simulink model "CM510A_MotAg3Meas"  (R2013b)
settings: Solver=FixedStepDiscrete  SolverMode=SingleTasking  StartTime=0.0  StopTime=1  FixedStep=0.0000625  RelTol=1e-3
values from neighbouring files (symbols this model uses):
  MOTAGCNTRREGMASK_CNT_U16 = DataDict.Constant    [CM510A_MotAg3Meas_DataDict.m]
  MOTAGLIM_CNT_U16 = DataDict.Constant    [CM510A_MotAg3Meas_DataDict.m]
undefined symbols (not defined in the file or in its folder): sigbuilder_block
libraries: simulink x4, NexteerUtilities x1
settings Model: RequirementInfo="{}  %GIDa_ca294f38_ed7c_4fb9_8c54_f4d56271bfc7"  ModifiedHistory=Rev 008: Updated model to Matlab 2013B, added comments to show requirement linkage  PauseTimes=0.5  Creator=nz3zln  LastModifiedBy=TZ8CY0
settings SolverCC: AutoInsertRateTranBlk=on  InsertRTBMode=Always
settings DataIOCC: LimitDataPoints=off  SaveFormat=Structure  ReturnWorkspaceOutputs=on
settings OptimizationCC: BlockReduction=off  InlineParams=on  ZeroExternalMemoryAtStartup=off  ZeroInternalMemoryAtStartup=off  OptimizeModelRefInitCode=on  LifeSpan=1
settings DebuggingCC: SignalInfNanChecking=error  SignalRangeChecking=warning  UnderspecifiedInitializationDetection=Simplified  SolverPrmCheckMsg=error  InheritedTsInSrcMsg=error  DiscreteInheritContinuousMsg=error  SingleTaskRateTransMsg=error  TasksWithSamePriorityMsg=error  SigSpecEnsureSampleTimeMsg=error  CheckMatrixSingularityMsg=error  ParameterUnderflowMsg=error  ParameterPrecisionLossMsg=error  ParameterTunabilityLossMsg=error  FixptConstUnderflowMsg=warning  FixptConstOverflowMsg=warning  VectorMatrixConversionMsg=error  SignalLabelMismatchMsg=error  UnconnectedInputMsg=error  UnconnectedOutputMsg=error  UnconnectedLineMsg=error  SFcnCompatibilityMsg=error  UniqueDataStoreMsg=warning  BusObjectLabelMismatch=error  RootOutportRequireBusObject=error  AssertControl=DisableAll  ModelReferenceIOMsg=error  ModelReferenceVersionMismatchMessage=warning  ModelReferenceIOMismatchMessage=error  ModelReferenceCSMismatchMessage=warning  ModelReferenceDataLoggingMessage=error  StateNameClashWarn=warning  StrictBusMsg=ErrorOnBusTreatedAsVector  NonBusSignalsTreatedAsBus=error  SFUnexpectedBacktrackingDiag=error  SFInvalidInputDataAccessInChartInitDiag=error  SFNoUnconditionalDefaultTransitionDiag=error  SFTransitionOutsideNaturalParentDiag=error  SFUnconditionalTransitionShadowingDiag=error  SFUndirectedBroadcastEventsDiag=error
settings ModelReferenceCC: ModelReferenceNumInstancesAllowed=Single
settings RTWCC: SystemTargetFile=autosar.tlc  GenCodeOnly=on  TemplateMakefile=ert_default_tmf  Description=AUTOSAR  GenerateReport=on  ProcessScript=autosar_make_rtw_hook  LaunchReport=on
settings CodeAppCC: GenerateComments=off  IgnoreCustomStorageClasses=off  CustomSymbolStrType=$N$R$M  CustomSymbolStrBlkIO=$N$M  SimulinkBlockComments=off
settings STFCustomTargetCC: ParMdlRefBuildCompliant=on  CompOptLevelCompliant=on  IncludeMdlTerminateFcn=off  CombineOutputUpdateFcns=on  SuppressErrorStatus=on  ERTFirstTimeCompliant=on  ERTCustomFileBanners=on  SupportNonFinite=off  SupportComplex=off  SupportContinuousTime=off  SupportNonInlinedSFcns=off  MATLABClassNameForMDSCustomization=Simulink.SoftwareTarget.ERTCustomization  AutosarCompliant=on  GRTInterface=off  SystemTargetFile=autosar.tlc
settings ERTTargetCC: CodeReplacementLibrary=ANSI_C  ConcurrentExecutionCompliant=off  IncludeMdlTerminateFcn=off  SuppressErrorStatus=on  SupportNonFinite=off  SupportComplex=off  ModelStepFunctionPrototypeControlCompliant=off  CPPClassGenCompliant=off  AutosarCompliant=on  InlinedParameterPlacement=NonHierarchical  ERTCustomFileTemplate=example_file_process.tlc  EnableUserReplacementTypes=on

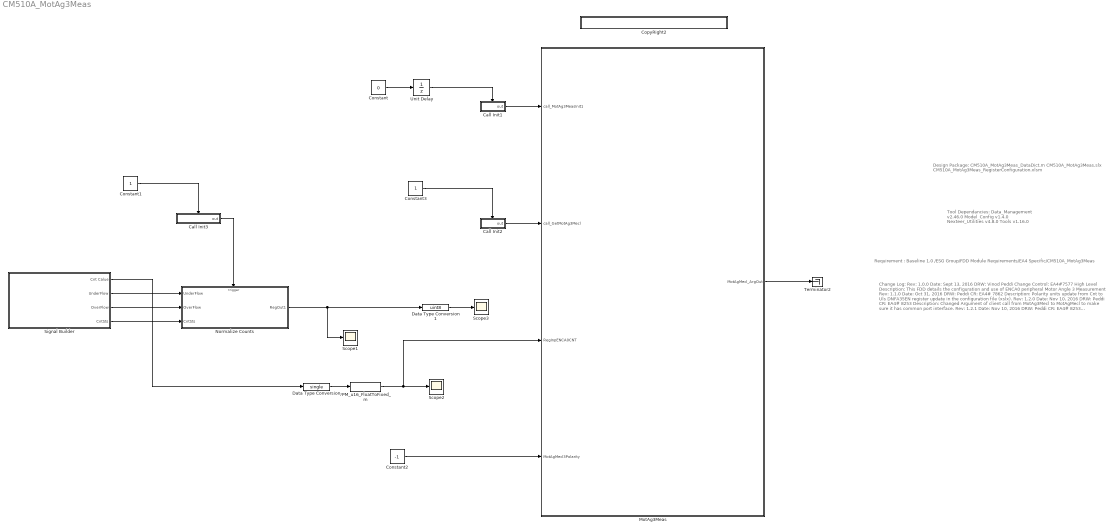
== system CM510A_MotAg3Meas ==
  note: Requirement : Baseline 1.0
      | /ESG Group/FDD Module Requirements/EA4 Specific/CM510A_MotAg3Meas
  note: Tool Dependancies:
      | Data_Management v2.46.0
      | Model_Config v1.4.0
      | Nexteer_Utilities v4.8.0
      | Tools v1.16.0
  note: Design Package:
      | CM510A_MotAg3Meas_DataDict.m
      | CM510A_MotAg3Meas.slx
      | CM510A_MotAg3Meas_RegisterConfiguration.xlsm
  note: Change Log:
      |
      | Rev: 1.0.0
      | Date: Sept 13, 2016
      | DRW: Vinod Peddi
      | Change Control: EA4#7577
      | High Level Description:
      | This FDD details the configuration and use of ENCA0 peripheral Motor Angle 3 Measurement
      |
      | Rev: 1.1.0
      | Date: Oct 31, 2016
      | DRW: Peddi
      | CR: EA4# 7862
      | Description: Polarity units update from Cnt to Uls
      | DNFA35EN register update in the configuration file (xslx).
      |
      | Rev: 1.2.0
      | Date: Nov 10, 2016
      | DRW: Peddi
      | CR: EA4# 8253
      | Description: Changed Argument of client call from MotAg3Mecl to MotAgMecl to
      | make sure it has common port interface.
      |
      | Rev: 1.2.1
      | Date: Nov 10, 2016
      | DRW: Peddi
      | CR: EA4# 8253
      | Description: Removed PIC and Noise Filter Config. (Will be handled by CM10)
  Call Init1 : Subsystem  TreatAsAtomicUnit=on
  Call Init2 : Subsystem  TreatAsAtomicUnit=on
  Call Init3 : Subsystem  TreatAsAtomicUnit=on
  Constant : Constant  Value=0  OutDataTypeStr=uint8
  Constant1 : Constant  OutDataTypeStr=int8
  Constant2 : Constant  Value=-1  OutDataTypeStr=int8
  Constant3 : Constant  OutDataTypeStr=int8
  CopyRight2 : Subsystem  Description=|  mask(Copyright Information){none=on}
      | Copyright info block.                                               
      |                                                                     
      | Place copyright information at the top of every subsystem in design.
      mask prompts: none "No parameters"
      mask help: Place copyright information at the top of every subsystem in design.
      mask Display:
      | NxtrConf = 'Nexteer Confidential';
      | 
      | sys = bdroot; %handle for the current model ("system")
      | first = get_param(sys,'Created');
      | first = first(end-3:end);  %year is last four digits
      | 
      | last = get_param(sys,'LastModifiedDate');
      | if isempty(last)
      |     last = datestr(now,'yyyy');
      | else
      |     last = last(end-3:end);
      | end
      | 
      | if strcmp(first,last)
      |     fprintf('%s -- Copyright %s Nexteer',NxtrConf,first)
      | else
      |     fprintf('%s -- %s%s- %s Nexteer',NxtrConf,char(169),first,last)
      | end
  Data Type Conversion : DataTypeConversion  OutDataTypeStr=single
  Data Type Conversion1 : DataTypeConversion  OutDataTypeStr=uint8
  FPM_u16_FloatToFixed_m : NexteerUtilities/Fixed Point Math Conversions/FPM_u16_FloatToFixed_m  SFunctionSpec=uint16 y1 = FPM_u16_FloatToFixed_m(single u1, single p1)  Param1=16
      settings: AttributesFormatString=u16_FloatToFixed
  MotAg3Meas : Subsystem
  Normalize Counts : Subsystem
  Scope1 : Scope
  Scope2 : Scope
      settings: SaveName=ScopeData7
  Scope3 : Scope
  Signal Builder : Subsystem  Tag=STV Subsys  LoadFcn=sigbuilder_block('load');  StartFcn=sigbuilder_block('start');  StopFcn=sigbuilder_block('stop');  ClipboardFcn=sigbuilder_block('clipboard');  mask(Sigbuilder block){}
      mask help: Simulink:masks:SigbuilderBlock_MD
      mask init:
      | if ~strcmp(get_param(bdroot(gcbh),'SimulationStatus'),'stopped') tuvar = sigbuilder_block('maskInit'); end
      settings: CopyFcn=sigbuilder_block('copy');  DeleteFcn=sigbuilder_block('delete');  ModelCloseFcn=sigbuilder_block('modelClose');  PreSaveFcn=sigbuilder_block('preSave');  PauseFcn=sigbuilder_block('pause');  ContinueFcn=sigbuilder_block('continue');  NameChangeFcn=sigbuilder_block('namechange');  OpenFcn=sigbuilder_block('open',[0 30 1440 723 ]);  CloseFcn=sigbuilder_block('close');
      mask Display: plot(0, 0, 100, 100,[2, 2, 32, 32, 2], [68, 8, 8, 68, 68],[32, 2], [38, 38], [32, 19, 2],[53, 60, 44], [32, 17, 17, 2],[16, 16, 31, 31]);txt = getActiveGroup(gcbh);text(2, 100, txt,'verticalAlignment', 'top');
  Terminator2 : Terminator
  Unit Delay : UnitDelay  InitialCondition=1  SampleTime=-1
  wires:
  Constant/1 -> Unit Delay/1
  Unit Delay/1 -> Call Init1/Enable
  Constant3/1 -> Call Init2/Enable
  Call Init1/1(out) -> MotAg3Meas/1(call_MotAg3MeasInit1)
  Call Init2/1(out) -> MotAg3Meas/2(call_GetMotAg3Mecl)
  FPM_u16_FloatToFixed_m/1 -> MotAg3Meas/3(RegInpENCA0CNT), Scope2/1
  Normalize Counts/1(RegOut1) -> Data Type Conversion1/1, Scope1/1
  MotAg3Meas/1(MotAgMecl_ArgOut) -> Terminator2/1
  Data Type Conversion/1 -> FPM_u16_FloatToFixed_m/1
  Constant1/1 -> Call Init3/Enable
  Call Init3/1(out) -> Normalize Counts/Trigger
  Signal Builder/1(Cnt Calue) -> Data Type Conversion/1
  Signal Builder/2(UnderFlow) -> Normalize Counts/1(UnderFlow)
  Signal Builder/3(OverFlow) -> Normalize Counts/2(OverFlow)
  Signal Builder/4(CntSts) -> Normalize Counts/3(CntSts)
  Data Type Conversion1/1 -> Scope3/1
  Constant2/1 -> MotAg3Meas/4(MotAgMecl3Polarity)

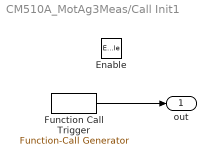
== system CM510A_MotAg3Meas/Call Init1 ==
  Enable : EnablePort
  Function Call Trigger : simulink/Ports & Subsystems/Function-Call Generator  RequirementInfo={} %GIDa_b7229461_487a_40de_bfdf_dab388053d82  sample_time=0.002  numberOfIterations=1
  out : Outport
  wires:
  Function Call Trigger/1 -> out/1

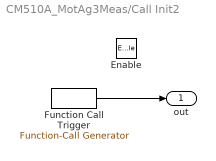
== system CM510A_MotAg3Meas/Call Init2 ==
  Enable : EnablePort
  Function Call Trigger : simulink/Ports & Subsystems/Function-Call Generator  RequirementInfo={} %GIDa_a0a97c4f_3e8f_431b_a781_191ff84f73ef  sample_time=0.0005  numberOfIterations=1
  out : Outport
  wires:
  Function Call Trigger/1 -> out/1

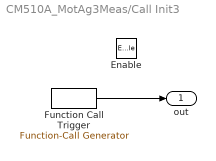
== system CM510A_MotAg3Meas/Call Init3 ==
  Enable : EnablePort
  Function Call Trigger : simulink/Ports & Subsystems/Function-Call Generator  RequirementInfo={} %GIDa_a0a97c4f_3e8f_431b_a781_191ff84f73ef  sample_time=0.0005  numberOfIterations=1
  out : Outport
  wires:
  Function Call Trigger/1 -> out/1

== system CM510A_MotAg3Meas/CopyRight2 ==

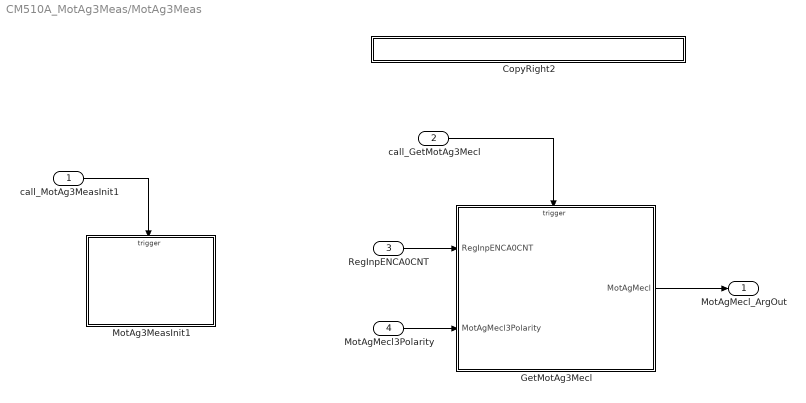
== system CM510A_MotAg3Meas/MotAg3Meas ==
  call_MotAg3MeasInit1 : Inport  RequirementInfo={} %GIDa_3f2124e9_01f6_42c8_98ca_c09f4c17d99d
  call_GetMotAg3Mecl : Inport  RequirementInfo={} %GIDa_a9829b41_47bf_4b01_8e96_1bb4faec4565  Port=2
  RegInpENCA0CNT : Inport  Port=3
  MotAgMecl3Polarity : Inport  Port=4
  CopyRight2 : Subsystem  Description=|  mask(Copyright Information){none=on}
      | Copyright info block.                                               
      |                                                                     
      | Place copyright information at the top of every subsystem in design.
      mask prompts: none "No parameters"
      mask help: Place copyright information at the top of every subsystem in design.
      mask Display:
      | NxtrConf = 'Nexteer Confidential';
      | 
      | sys = bdroot; %handle for the current model ("system")
      | first = get_param(sys,'Created');
      | first = first(end-3:end);  %year is last four digits
      | 
      | last = get_param(sys,'LastModifiedDate');
      | if isempty(last)
      |     last = datestr(now,'yyyy');
      | else
      |     last = last(end-3:end);
      | end
      | 
      | if strcmp(first,last)
      |     fprintf('%s -- Copyright %s Nexteer',NxtrConf,first)
      | else
      |     fprintf('%s -- %s%s- %s Nexteer',NxtrConf,char(169),first,last)
      | end
  GetMotAg3Mecl : Subsystem  RequirementInfo="{'linktype_rmi_doors' '00011b4f (/ESG Group/FDD Module Requirements/EA4 Specific/CM510A_MotAg3Meas)' '#CM510A_15' 'true' 'REQ:  CM510A_15' '' } %GIDa_dbd08618_b447_4b13_a314_37af3685d10a"
  MotAg3MeasInit1 : Subsystem
  MotAgMecl_ArgOut : Outport
  wires:
  call_MotAg3MeasInit1/1 -> MotAg3MeasInit1/Trigger
  call_GetMotAg3Mecl/1 -> GetMotAg3Mecl/Trigger
  RegInpENCA0CNT/1 -> GetMotAg3Mecl/1(RegInpENCA0CNT)
  GetMotAg3Mecl/1(MotAgMecl) -> MotAgMecl_ArgOut/1
  MotAgMecl3Polarity/1 -> GetMotAg3Mecl/2(MotAgMecl3Polarity)

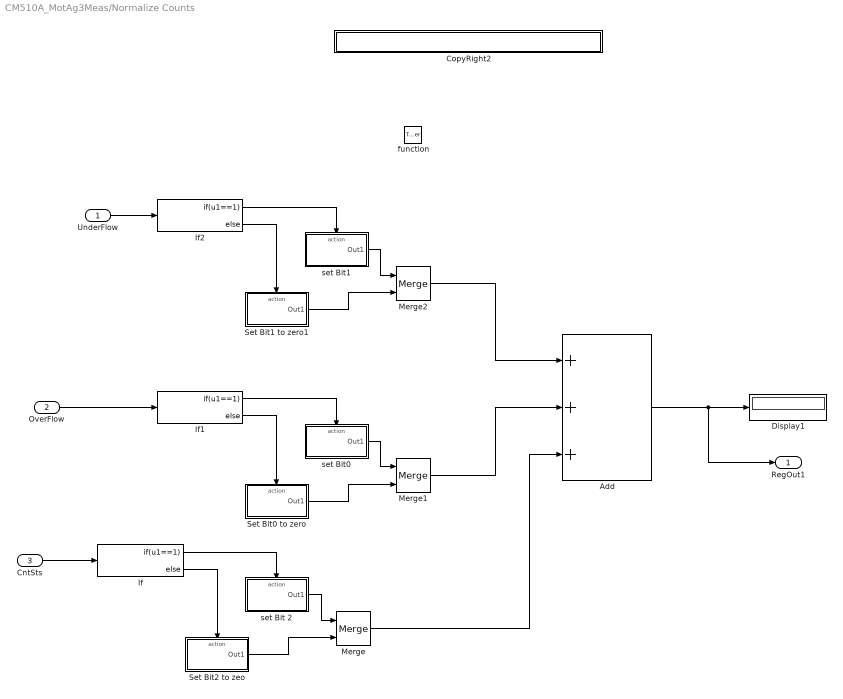
== system CM510A_MotAg3Meas/Normalize Counts ==
  UnderFlow : Inport
  OverFlow : Inport  Port=2
  CntSts : Inport  Port=3
  function : TriggerPort  TriggerType=function-call
  Add : Sum  Inputs=+++
  CopyRight2 : Subsystem  Description=|  mask(Copyright Information){none=on}
      | Copyright info block.                                               
      |                                                                     
      | Place copyright information at the top of every subsystem in design.
      mask prompts: none "No parameters"
      mask help: Place copyright information at the top of every subsystem in design.
      mask Display:
      | NxtrConf = 'Nexteer Confidential';
      | 
      | sys = bdroot; %handle for the current model ("system")
      | first = get_param(sys,'Created');
      | first = first(end-3:end);  %year is last four digits
      | 
      | last = get_param(sys,'LastModifiedDate');
      | if isempty(last)
      |     last = datestr(now,'yyyy');
      | else
      |     last = last(end-3:end);
      | end
      | 
      | if strcmp(first,last)
      |     fprintf('%s -- Copyright %s Nexteer',NxtrConf,first)
      | else
      |     fprintf('%s -- %s%s- %s Nexteer',NxtrConf,char(169),first,last)
      | end
  Display1 : Display
  If : If  IfExpression=u1==1
  If1 : If  IfExpression=u1==1
  If2 : If  IfExpression=u1==1
  Merge : Merge
  Merge1 : Merge
  Merge2 : Merge
  Set Bit0 to zero : Subsystem  TreatAsAtomicUnit=on
  Set Bit1 to zero1 : Subsystem  TreatAsAtomicUnit=on
  Set Bit2 to zeo : Subsystem  TreatAsAtomicUnit=on
  set Bit 2 : Subsystem  TreatAsAtomicUnit=on
  set Bit0 : Subsystem  TreatAsAtomicUnit=on
  set Bit1 : Subsystem  TreatAsAtomicUnit=on
  RegOut1 : Outport
  wires:
  CntSts/1 -> If/1
  If/1 -> set Bit 2/Action
  If/2 -> Set Bit2 to zeo/Action
  set Bit 2/1(Out1) -> Merge/1
  Set Bit2 to zeo/1(Out1) -> Merge/2
  If1/1 -> set Bit0/Action
  If1/2 -> Set Bit0 to zero/Action
  set Bit0/1(Out1) -> Merge1/1
  Set Bit0 to zero/1(Out1) -> Merge1/2
  OverFlow/1 -> If1/1
  If2/1 -> set Bit1/Action
  If2/2 -> Set Bit1 to zero1/Action
  set Bit1/1(Out1) -> Merge2/1
  Set Bit1 to zero1/1(Out1) -> Merge2/2
  UnderFlow/1 -> If2/1
  Merge2/1 -> Add/1
  Merge1/1 -> Add/2
  Merge/1 -> Add/3
  Add/1 -> RegOut1/1, Display1/1

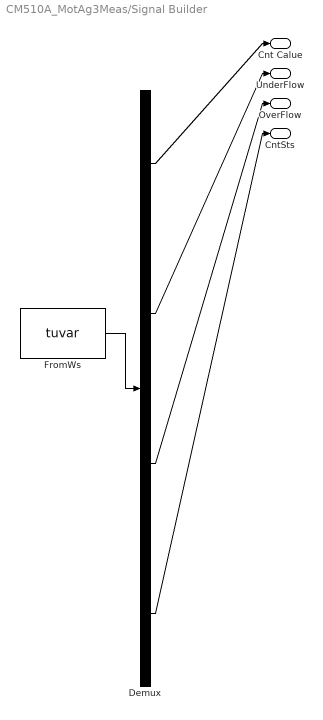
== system CM510A_MotAg3Meas/Signal Builder ==
  Demux : Demux  Tag=STV Demux
  FromWs : FromWorkspace  Tag=STV FromWs  VariableName=tuvar  SampleTime=0
      SigBuilderData=|
      | common.afterFinalStr = 'Extrapolate'
      | common.sampleTime = 0
      | dataSet(1).timeRange = [0 1]
      | dataSet(1).name = 'UpCount'
      | dataSet(2).timeRange = [0 1]
      | dataSet(2).name = 'DownCount'
      | sbobj.Groups(1).Name = 'UpCount'
      | sbobj.Groups(1).Signals(1).Name = 'Cnt Calue'
      | sbobj.Groups(1).Signals(1).XData = [0 0.2 0.2 0.3 0.4 0.4 0.6 1]
      | sbobj.Groups(1).Signals(1).YData = [0 1 0 0.5 0 1 0 1]
      | sbobj.Groups(1).Signals(2).Name = 'UnderFlow'
      | sbobj.Groups(1).Signals(2).XData = [0 0.5 1]
      | sbobj.Groups(1).Signals(2).YData = [0 0 0]
      | sbobj.Groups(1).Signals(3).Name = 'OverFlow'
      | sbobj.Groups(1).Signals(3).XData = [0 0.499 0.499 0.5 0.5 1]
      | sbobj.Groups(1).Signals(3).YData = [0 0 1 1 0 0]
      | sbobj.Groups(1).Signals(4).Name = 'CntSts'
      | sbobj.Groups(1).Signals(4).XData = [0 1]
      | sbobj.Groups(1).Signals(4).YData = [0 0]
      | sbobj.Groups(1).TimeRange = [0 1]
      | sbobj.Groups(2).Name = 'DownCount'
      | sbobj.Groups(2).Signals(1).Name = 'Cnt Calue'
      | sbobj.Groups(2).Signals(1).XData = [0 1]
      | sbobj.Groups(2).Signals(1).YData = [1 0]
      | sbobj.Groups(2).Signals(2).Name = 'UnderFlow'
      | sbobj.Groups(2).Signals(2).XData = [0 0.499 0.499 0.5 0.5 1]
      | sbobj.Groups(2).Signals(2).YData = [0 0 1 1 0 0]
      | sbobj.Groups(2).Signals(3).Name = 'OverFlow'
      | sbobj.Groups(2).Signals(3).XData = [0 1]
      | sbobj.Groups(2).Signals(3).YData = [0 0]
      | sbobj.Groups(2).Signals(4).Name = 'CntSts'
      | sbobj.Groups(2).Signals(4).XData = [0 1]
      | sbobj.Groups(2).Signals(4).YData = [1 1]
      | sbobj.Groups(2).TimeRange = [0 1]
  Cnt Calue : Outport  Tag=STV Outport
  UnderFlow : Outport  Tag=STV Outport  Port=2
  OverFlow : Outport  Tag=STV Outport  Port=3
  CntSts : Outport  Tag=STV Outport  Port=4
  wires:
  FromWs/1 -> Demux/1
  Demux/1 -> Cnt Calue/1
  Demux/2 -> UnderFlow/1
  Demux/3 -> OverFlow/1
  Demux/4 -> CntSts/1

== system CM510A_MotAg3Meas/MotAg3Meas/CopyRight2 ==

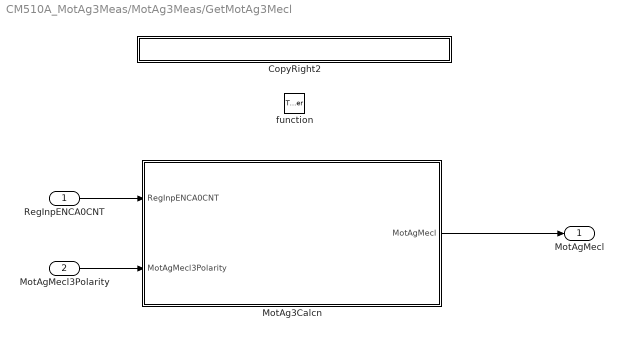
== system CM510A_MotAg3Meas/MotAg3Meas/GetMotAg3Mecl ==
  RegInpENCA0CNT : Inport
  MotAgMecl3Polarity : Inport  Port=2
  function : TriggerPort  TriggerType=function-call
  CopyRight2 : Subsystem  Description=|  mask(Copyright Information){none=on}
      | Copyright info block.                                               
      |                                                                     
      | Place copyright information at the top of every subsystem in design.
      mask prompts: none "No parameters"
      mask help: Place copyright information at the top of every subsystem in design.
      mask Display:
      | NxtrConf = 'Nexteer Confidential';
      | 
      | sys = bdroot; %handle for the current model ("system")
      | first = get_param(sys,'Created');
      | first = first(end-3:end);  %year is last four digits
      | 
      | last = get_param(sys,'LastModifiedDate');
      | if isempty(last)
      |     last = datestr(now,'yyyy');
      | else
      |     last = last(end-3:end);
      | end
      | 
      | if strcmp(first,last)
      |     fprintf('%s -- Copyright %s Nexteer',NxtrConf,first)
      | else
      |     fprintf('%s -- %s%s- %s Nexteer',NxtrConf,char(169),first,last)
      | end
  MotAg3Calcn : Subsystem
  MotAgMecl : Outport
  wires:
  RegInpENCA0CNT/1 -> MotAg3Calcn/1(RegInpENCA0CNT)
  MotAg3Calcn/1(MotAgMecl) -> MotAgMecl/1
  MotAgMecl3Polarity/1 -> MotAg3Calcn/2(MotAgMecl3Polarity)

== system CM510A_MotAg3Meas/MotAg3Meas/MotAg3MeasInit1 ==
  function : TriggerPort  TriggerType=function-call
  CopyRight2 : Subsystem  Description=|  mask(Copyright Information){none=on}
      | Copyright info block.                                               
      |                                                                     
      | Place copyright information at the top of every subsystem in design.
      mask prompts: none "No parameters"
      mask help: Place copyright information at the top of every subsystem in design.
      mask Display:
      | NxtrConf = 'Nexteer Confidential';
      | 
      | sys = bdroot; %handle for the current model ("system")
      | first = get_param(sys,'Created');
      | first = first(end-3:end);  %year is last four digits
      | 
      | last = get_param(sys,'LastModifiedDate');
      | if isempty(last)
      |     last = datestr(now,'yyyy');
      | else
      |     last = last(end-3:end);
      | end
      | 
      | if strcmp(first,last)
      |     fprintf('%s -- Copyright %s Nexteer',NxtrConf,first)
      | else
      |     fprintf('%s -- %s%s- %s Nexteer',NxtrConf,char(169),first,last)
      | end
  Initialize ENCA Registers : Subsystem  TreatAsAtomicUnit=on

== system CM510A_MotAg3Meas/Normalize Counts/CopyRight2 ==

== system CM510A_MotAg3Meas/Normalize Counts/Set Bit0 to zero ==
  Action Port : ActionPort  ActionType=else
  Constant : Constant  Value=0  OutDataTypeStr=uint8
  Out1 : Outport
  wires:
  Constant/1 -> Out1/1

== system CM510A_MotAg3Meas/Normalize Counts/Set Bit1 to zero1 ==
  Action Port : ActionPort  ActionType=else
  Constant : Constant  Value=0  OutDataTypeStr=uint8
  Out1 : Outport
  wires:
  Constant/1 -> Out1/1

== system CM510A_MotAg3Meas/Normalize Counts/Set Bit2 to zeo ==
  Action Port : ActionPort  ActionType=else
  Constant : Constant  Value=0  OutDataTypeStr=uint8
  Out1 : Outport
  wires:
  Constant/1 -> Out1/1

== system CM510A_MotAg3Meas/Normalize Counts/set Bit 2 ==
  Action Port : ActionPort  ActionType=then
  Constant : Constant  Value=4  OutDataTypeStr=uint8
  Out1 : Outport
  wires:
  Constant/1 -> Out1/1

== system CM510A_MotAg3Meas/Normalize Counts/set Bit0 ==
  Action Port : ActionPort  ActionType=then
  Constant : Constant  OutDataTypeStr=uint8
  Out1 : Outport
  wires:
  Constant/1 -> Out1/1

== system CM510A_MotAg3Meas/Normalize Counts/set Bit1 ==
  Action Port : ActionPort  ActionType=then
  Constant : Constant  Value=2  OutDataTypeStr=uint8
  Out1 : Outport
  wires:
  Constant/1 -> Out1/1

== system CM510A_MotAg3Meas/MotAg3Meas/GetMotAg3Mecl/CopyRight2 ==

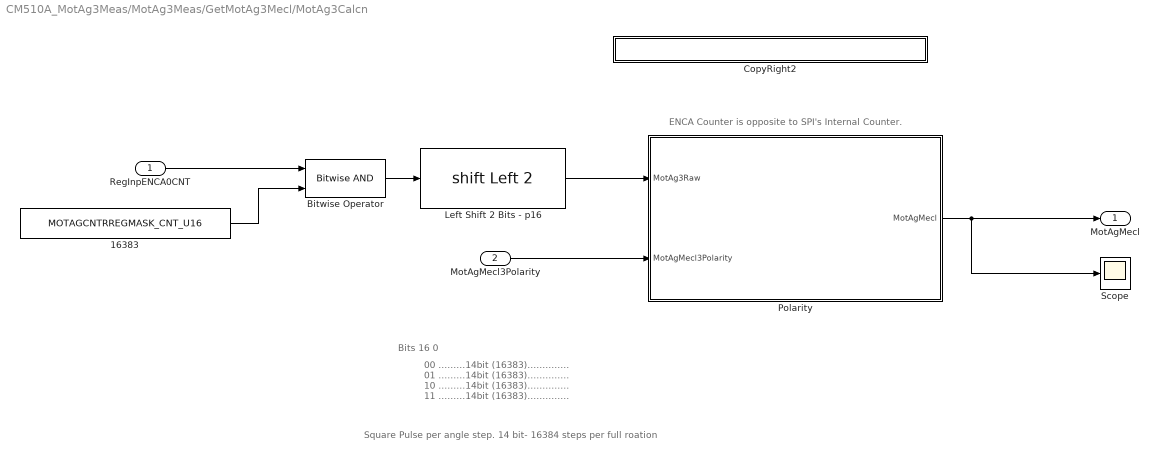
== system CM510A_MotAg3Meas/MotAg3Meas/GetMotAg3Mecl/MotAg3Calcn ==
  note: Square Pulse per angle step. 14 bit- 16384 steps per full roation
  note: ENCA Counter is opposite to SPI's Internal Counter.
  note: Bits 16 0
  note: 00 .........14bit (16383)..............
      | 01 .........14bit (16383)..............
      | 10 .........14bit (16383)..............
      | 11 .........14bit (16383)..............
  RegInpENCA0CNT : Inport  RequirementInfo="{'linktype_rmi_doors' '00011b4f (/ESG Group/FDD Module Requirements/EA4 Specific/CM510A_MotAg3Meas)' '#CM510A_66' 'true' 'REQ:  CM510A_66' '' } %GIDa_08ec8d51_6bf0_485e_bf0c_e07448ca5708"
  MotAgMecl3Polarity : Inport  RequirementInfo="{'linktype_rmi_doors' '00011b4f (/ESG Group/FDD Module Requirements/EA4 Specific/CM510A_MotAg3Meas)' '#CM510A_67' 'true' 'REQ:  CM510A_67' '' } %GIDa_a154c5c1_f9bb_4438_a4db_c13dbdf13071"  Port=2
  16383 : Constant  RequirementInfo="{'linktype_rmi_doors' '00011b4f (/ESG Group/FDD Module Requirements/EA4 Specific/CM510A_MotAg3Meas)' '#CM510A_66' 'true' 'REQ:  CM510A_66' '' } %GIDa_c0dd3f32_81e1_4d09_b8fe_2e8838c8b21c"  Value=MOTAGCNTRREGMASK_CNT_U16
  Bitwise Operator : simulink/Logic and Bit Operations/Bitwise Operator  RequirementInfo="{'linktype_rmi_doors' '00011b4f (/ESG Group/FDD Module Requirements/EA4 Specific/CM510A_MotAg3Meas)' '#CM510A_66' 'true' 'REQ:  CM510A_66' '' } %GIDa_a2bf002a_d1f5_43d9_b1cc_8ae2bafc417c"  logicop=AND  UseBitMask=off  NumInputPorts=2  BitMask=16383  BitMaskRealWorld=Stored Integer
  CopyRight2 : Subsystem  Description=|  mask(Copyright Information){none=on}
      | Copyright info block.                                               
      |                                                                     
      | Place copyright information at the top of every subsystem in design.
      mask prompts: none "No parameters"
      mask help: Place copyright information at the top of every subsystem in design.
      mask Display:
      | NxtrConf = 'Nexteer Confidential';
      | 
      | sys = bdroot; %handle for the current model ("system")
      | first = get_param(sys,'Created');
      | first = first(end-3:end);  %year is last four digits
      | 
      | last = get_param(sys,'LastModifiedDate');
      | if isempty(last)
      |     last = datestr(now,'yyyy');
      | else
      |     last = last(end-3:end);
      | end
      | 
      | if strcmp(first,last)
      |     fprintf('%s -- Copyright %s Nexteer',NxtrConf,first)
      | else
      |     fprintf('%s -- %s%s- %s Nexteer',NxtrConf,char(169),first,last)
      | end
  Left Shift 2 Bits - p16 : ArithShift  RequirementInfo="{'linktype_rmi_doors' '00011b4f (/ESG Group/FDD Module Requirements/EA4 Specific/CM510A_MotAg3Meas)' '#CM510A_66' 'true' 'REQ:  CM510A_66' '' } %GIDa_e6c89e43_3576_4000_a35f_842f25e1a1b7"  BitShiftNumber=2  BitShiftDirection=Left
  Polarity : Subsystem  RequirementInfo="{'linktype_rmi_doors' '00011b4f (/ESG Group/FDD Module Requirements/EA4 Specific/CM510A_MotAg3Meas)' '#CM510A_67' 'true' 'REQ:  CM510A_67' '' } %GIDa_f744dcfa_c060_4788_aa5c_dd845431b195"
  Scope : Scope
      settings: SaveName=ScopeData5
  MotAgMecl : Outport
  wires:
  Polarity/1(MotAgMecl) -> Scope/1, MotAgMecl/1
  Bitwise Operator/1 -> Left Shift 2 Bits - p16/1
  Left Shift 2 Bits - p16/1 -> Polarity/1(MotAg3Raw)
  RegInpENCA0CNT/1 -> Bitwise Operator/1
  16383/1 -> Bitwise Operator/2
  MotAgMecl3Polarity/1 -> Polarity/2(MotAgMecl3Polarity)

== system CM510A_MotAg3Meas/MotAg3Meas/MotAg3MeasInit1/CopyRight2 ==

== system CM510A_MotAg3Meas/MotAg3Meas/MotAg3MeasInit1/Initialize ENCA Registers ==
  note: 1.  Configure the ENCA registers according to CM510A_MotAg3Meas_RegisterConfiguration.xlsm
      |     Order by Row.
  CopyRight2 : Subsystem  Description=|  mask(Copyright Information){none=on}
      | Copyright info block.                                               
      |                                                                     
      | Place copyright information at the top of every subsystem in design.
      mask prompts: none "No parameters"
      mask help: Place copyright information at the top of every subsystem in design.
      mask Display:
      | NxtrConf = 'Nexteer Confidential';
      | 
      | sys = bdroot; %handle for the current model ("system")
      | first = get_param(sys,'Created');
      | first = first(end-3:end);  %year is last four digits
      | 
      | last = get_param(sys,'LastModifiedDate');
      | if isempty(last)
      |     last = datestr(now,'yyyy');
      | else
      |     last = last(end-3:end);
      | end
      | 
      | if strcmp(first,last)
      |     fprintf('%s -- Copyright %s Nexteer',NxtrConf,first)
      | else
      |     fprintf('%s -- %s%s- %s Nexteer',NxtrConf,char(169),first,last)
      | end

== system CM510A_MotAg3Meas/MotAg3Meas/GetMotAg3Mecl/MotAg3Calcn/CopyRight2 ==

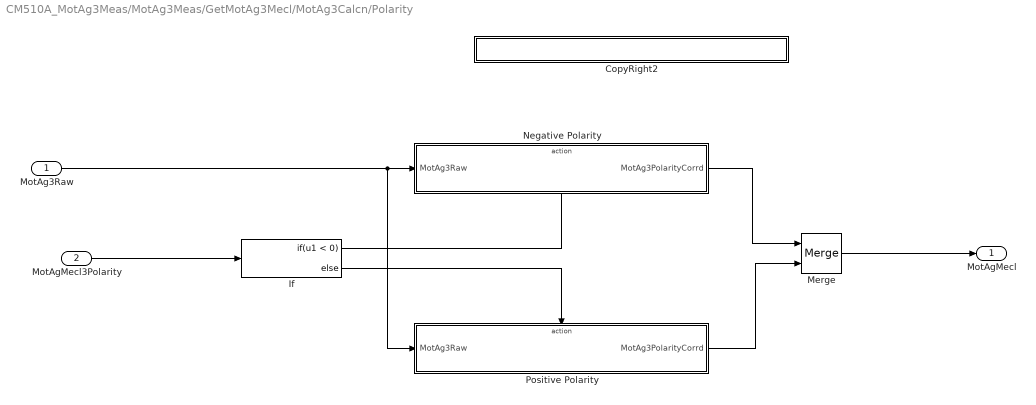
== system CM510A_MotAg3Meas/MotAg3Meas/GetMotAg3Mecl/MotAg3Calcn/Polarity ==
  MotAg3Raw : Inport
  MotAgMecl3Polarity : Inport  Port=2
  CopyRight2 : Subsystem  Description=|  mask(Copyright Information){none=on}
      | Copyright info block.                                               
      |                                                                     
      | Place copyright information at the top of every subsystem in design.
      mask prompts: none "No parameters"
      mask help: Place copyright information at the top of every subsystem in design.
      mask Display:
      | NxtrConf = 'Nexteer Confidential';
      | 
      | sys = bdroot; %handle for the current model ("system")
      | first = get_param(sys,'Created');
      | first = first(end-3:end);  %year is last four digits
      | 
      | last = get_param(sys,'LastModifiedDate');
      | if isempty(last)
      |     last = datestr(now,'yyyy');
      | else
      |     last = last(end-3:end);
      | end
      | 
      | if strcmp(first,last)
      |     fprintf('%s -- Copyright %s Nexteer',NxtrConf,first)
      | else
      |     fprintf('%s -- %s%s- %s Nexteer',NxtrConf,char(169),first,last)
      | end
  If : If  IfExpression=u1 < 0
  Merge : Merge
  Negative Polarity : Subsystem  TreatAsAtomicUnit=on
  Positive Polarity : Subsystem  TreatAsAtomicUnit=on
  MotAgMecl : Outport
  wires:
  MotAgMecl3Polarity/1 -> If/1
  MotAg3Raw/1 -> Positive Polarity/1(MotAg3Raw), Negative Polarity/1(MotAg3Raw)
  If/1 -> Negative Polarity/Action
  If/2 -> Positive Polarity/Action
  Negative Polarity/1(MotAg3PolarityCorrd) -> Merge/1
  Positive Polarity/1(MotAg3PolarityCorrd) -> Merge/2
  Merge/1 -> MotAgMecl/1

== system CM510A_MotAg3Meas/MotAg3Meas/MotAg3MeasInit1/Initialize ENCA Registers/CopyRight2 ==

== system CM510A_MotAg3Meas/MotAg3Meas/GetMotAg3Mecl/MotAg3Calcn/Polarity/CopyRight2 ==

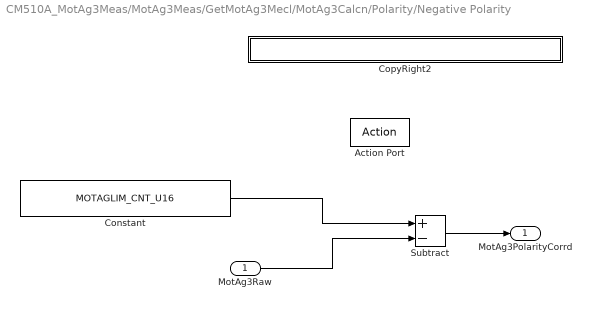
== system CM510A_MotAg3Meas/MotAg3Meas/GetMotAg3Mecl/MotAg3Calcn/Polarity/Negative Polarity ==
  MotAg3Raw : Inport
  Action Port : ActionPort  ActionType=then
  Constant : Constant  Value=MOTAGLIM_CNT_U16
  CopyRight2 : Subsystem  Description=|  mask(Copyright Information){none=on}
      | Copyright info block.                                               
      |                                                                     
      | Place copyright information at the top of every subsystem in design.
      mask prompts: none "No parameters"
      mask help: Place copyright information at the top of every subsystem in design.
      mask Display:
      | NxtrConf = 'Nexteer Confidential';
      | 
      | sys = bdroot; %handle for the current model ("system")
      | first = get_param(sys,'Created');
      | first = first(end-3:end);  %year is last four digits
      | 
      | last = get_param(sys,'LastModifiedDate');
      | if isempty(last)
      |     last = datestr(now,'yyyy');
      | else
      |     last = last(end-3:end);
      | end
      | 
      | if strcmp(first,last)
      |     fprintf('%s -- Copyright %s Nexteer',NxtrConf,first)
      | else
      |     fprintf('%s -- %s%s- %s Nexteer',NxtrConf,char(169),first,last)
      | end
  Subtract : Sum  Inputs=+-
  MotAg3PolarityCorrd : Outport
  wires:
  Constant/1 -> Subtract/1
  MotAg3Raw/1 -> Subtract/2
  Subtract/1 -> MotAg3PolarityCorrd/1

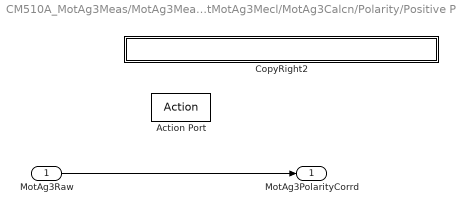
== system CM510A_MotAg3Meas/MotAg3Meas/GetMotAg3Mecl/MotAg3Calcn/Polarity/Positive Polarity ==
  MotAg3Raw : Inport
  Action Port : ActionPort  ActionType=else
  CopyRight2 : Subsystem  Description=|  mask(Copyright Information){none=on}
      | Copyright info block.                                               
      |                                                                     
      | Place copyright information at the top of every subsystem in design.
      mask prompts: none "No parameters"
      mask help: Place copyright information at the top of every subsystem in design.
      mask Display:
      | NxtrConf = 'Nexteer Confidential';
      | 
      | sys = bdroot; %handle for the current model ("system")
      | first = get_param(sys,'Created');
      | first = first(end-3:end);  %year is last four digits
      | 
      | last = get_param(sys,'LastModifiedDate');
      | if isempty(last)
      |     last = datestr(now,'yyyy');
      | else
      |     last = last(end-3:end);
      | end
      | 
      | if strcmp(first,last)
      |     fprintf('%s -- Copyright %s Nexteer',NxtrConf,first)
      | else
      |     fprintf('%s -- %s%s- %s Nexteer',NxtrConf,char(169),first,last)
      | end
  MotAg3PolarityCorrd : Outport
  wires:
  MotAg3Raw/1 -> MotAg3PolarityCorrd/1

== system CM510A_MotAg3Meas/MotAg3Meas/GetMotAg3Mecl/MotAg3Calcn/Polarity/Negative Polarity/CopyRight2 ==

== system CM510A_MotAg3Meas/MotAg3Meas/GetMotAg3Mecl/MotAg3Calcn/Polarity/Positive Polarity/CopyRight2 ==
